simulink model "lookupTableDynamic_TestGen5"  (R2017b)
settings: Solver=FixedStepDiscrete  StartTime=0.0  StopTime=10.0  RelTol=1e-3
libraries: simulink x1
settings Model: Creator=ktrinh  LastModifiedBy=ktrinh
settings DebuggingCC: ParameterOverflowMsg=none

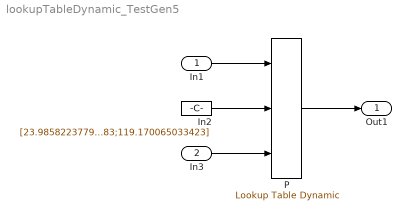
== system lookupTableDynamic_TestGen5 ==
  In1 : Inport  OutMin=21.9858  OutMax=121  OutDataTypeStr=int16  PortDimensions=1
  In3 : Inport  Port=2  PortDimensions=5
  In2 : Constant  Value=[23.9858223779924;89.0500675126042;92.0917415492865;102.002183808383;119.170065033423]  OutDataTypeStr=int16
  P : simulink/Lookup Tables/Lookup Table Dynamic  LookUpMeth=Interpolation-Extrapolation  OutDataType=fixdt('int16')  OutScaling=[]  OutputDataTypeScalingMode=Specify via dialog  OutDataTypeStr=int16  RndMeth=Simplest  DoSatur=on
      settings: SourceProductName=Simulink
  Out1 : Outport
  wires:
  In1/1 -> P/1
  In2/1 -> P/2
  In3/1 -> P/3
  P/1 -> Out1/1
